simulink model "modelerwin"  (R2014a)
settings: Solver=ode45  StartTime=0.0  StopTime=25  MaxStep=0.05  RelTol=1e-5
values from neighbouring files (symbols this model uses):
  A = [0,1;0,-1.782000000000000]    [ModelValues.m]    (also in modelerwin.mat = [-2.02973141125  0.612067387973; -0.07490477511  -2.45796858; newpoles.m = A_old2-B*K)
  B = [0;-39.940000000000000]    [ModelValues.m]    (also in modelerwin.mat = [2.4327 6.1289])
  C = [1,0]    [ModelValues.m]    (also in modelerwin.mat = [7.8178 -7.0269])
  InitalCond = [0 0]    [modelerwin.mat]
  K = acker(A, B, K_poles)    [ModelValues.m]    (also in modelerwin.mat = [-0.19331137779 -0.170019320147]; newpoles.m = acker(A_old2,B,poles))
  L = acker(A', C', L_poles)    [ModelValues.m]    (also in modelerwin.mat = [0.677100111676 0.253473544958]; newpoles.m = acker(A',C',Lpoles)')
  Nbar = -0.106325186801    [modelerwin.mat]    (also in newpoles.m = rscale(A,B,C,D,K))
libraries: simulink x1
settings Model: Creator=Erwin  LastModifiedBy=Erwin
settings SolverCC: ZeroCrossAlgorithm=Adaptive
settings DebuggingCC: SolverPrmCheckMsg=none

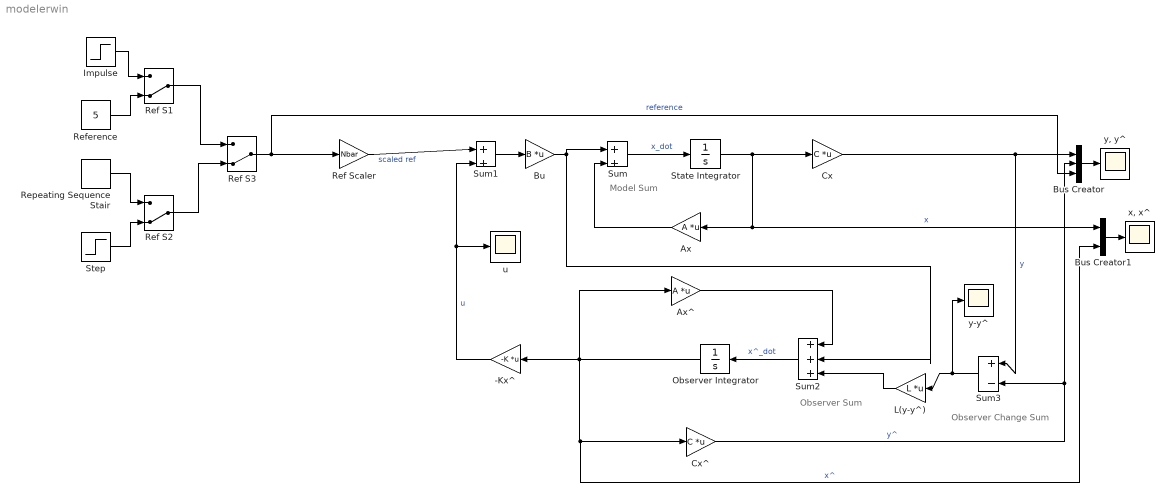
== system modelerwin ==
  note: Observer Change Sum
  note: Observer Sum
  note: Model Sum
  -Kx^ : Gain  Gain=-K  Multiplication=Matrix(K*u)
  Ax : Gain  Gain=A  Multiplication=Matrix(K*u)
  Ax^ : Gain  Gain=A  Multiplication=Matrix(K*u)
  Bu : Gain  Gain=B  Multiplication=Matrix(K*u)
  Bus Creator : BusCreator  Inputs=3
  Bus Creator1 : BusCreator  Inputs=2
  Cx : Gain  Gain=C  Multiplication=Matrix(K*u)
  Cx^ : Gain  Gain=C  Multiplication=Matrix(K*u)
  Impulse : Step  Time=0.001  Before=10  After=0  SampleTime=0
  L(y-y^) : Gain  Gain=L  Multiplication=Matrix(K*u)
  Observer Integrator : Integrator  InitialCondition=InitalCond  ContinuousStateAttributes=['position';'velocity']
  Ref S1 : ManualSwitch  CurrentSetting=0
  Ref S2 : ManualSwitch  CurrentSetting=0
  Ref S3 : ManualSwitch  CurrentSetting=0
  Ref Scaler : Gain  Gain=Nbar
  Reference : Constant  Value=5
  Repeating Sequence Stair : simulink/Sources/Repeating Sequence Stair  OutValues=[5 -5 10 -10 0].'  tsamp=5  OutMin=[]  OutMax=[]  OutDataTypeStr=double  OutputDataTypeScalingMode=double  OutDataType=fixdt(0,8)  ConRadixGroup=Best Precision: Vector-wise  OutScaling=2^-12
  State Integrator : Integrator  InitialCondition=InitalCond  ContinuousStateAttributes=['position';'velocity']
  Step : Step  After=10  SampleTime=0
  Sum : Sum  Inputs=|++
  Sum1 : Sum  Inputs=|++
  Sum2 : Sum  Inputs=|+++
  Sum3 : Sum  Inputs=|+-
  u : Scope
      settings: ShowLegends=on  SaveName=ScopeData3
  "x, x^" : Scope
      settings: ShowLegends=on
  "y, y^" : Scope
      settings: ShowLegends=on
  y-y^ : Scope
      settings: SaveName=ScopeData2
  wires:
  State Integrator/1 -> Cx/1, Bus Creator1/1, Ax/1  "x"
  Sum/1 -> State Integrator/1  "x_dot"
  Ax/1 -> Sum/2
  Bu/1 -> Sum2/2, Sum/1
  Cx/1 -> Bus Creator/1, Sum3/1  "y"
  Observer Integrator/1 -> Bus Creator1/2, Cx^/1, Ax^/1, -Kx^/1  "x^"
  Sum2/1 -> Observer Integrator/1  "x^_dot"
  Ax^/1 -> Sum2/1
  Sum3/1 -> y-y^/1, L(y-y^)/1
  Cx^/1 -> Bus Creator/2, Sum3/2  "y^"
  L(y-y^)/1 -> Sum2/3
  Bus Creator/1 -> "y, y^"/1
  Bus Creator1/1 -> "x, x^"/1
  Sum1/1 -> Bu/1
  -Kx^/1 -> u/1, Sum1/2  "u"
  Ref S3/1 -> Ref Scaler/1, Bus Creator/3  "reference"
  Reference/1 -> Ref S1/2
  Repeating Sequence Stair/1 -> Ref S2/1
  Step/1 -> Ref S2/2
  Ref S2/1 -> Ref S3/2
  Ref Scaler/1 -> Sum1/1  "scaled ref"
  Impulse/1 -> Ref S1/1
  Ref S1/1 -> Ref S3/1
